simulink model "model1_raw"  (Simulink 7.7)
settings: Solver=VariableStepDiscrete  StartTime=0.0  StopTime=10.0  RelTol=1e-3
values from neighbouring files (symbols this model uses):
  A = A1'    [dyskretny.m]    (also in przebieg.m; zmiennestanu.m)
  C = B1'    [dyskretny.m]    (also in przebieg.m; zmiennestanu.m)
libraries: simulink x3
settings Model: Creator=Andones  LastModifiedBy=qiubix

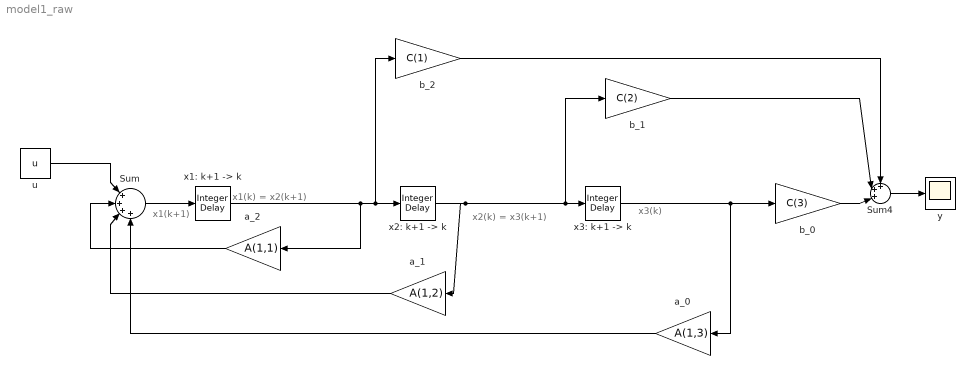
== system model1_raw ==
  note: x1(k+1)
  note: x3(k)
  note: x1(k) = x2(k+1)
  note: x2(k) = x3(k+1)
  " x3: k+1 -> k" : simulink/Discrete/Integer Delay  NumDelays=1  vinit=1  samptime=T_s
  Sum : Sum  Inputs=|++++
  Sum4 : Sum  Inputs=+++|
  a_0 : Gain  Gain=A(1,3)
  a_1 : Gain  Gain=A(1,2)
  a_2 : Gain  Gain=A(1,1)
  b_0 : Gain  Gain=C(3)
  b_1 : Gain  Gain=C(2)
  b_2 : Gain  Gain=C(1)
  u : Constant  Value=u
  "x1: k+1 -> k " : simulink/Discrete/Integer Delay  NumDelays=1  vinit=-1  samptime=T_s
  "x2: k+1 -> k" : simulink/Discrete/Integer Delay  NumDelays=1  vinit=-1  samptime=T_s
  y : Scope
  wires:
  Sum/1 -> "x1: k+1 -> k "/1
  Sum4/1 -> y/1
  b_0/1 -> Sum4/3
  b_1/1 -> Sum4/2
  b_2/1 -> Sum4/1
  "x1: k+1 -> k "/1 -> "x2: k+1 -> k"/1, b_2/1, a_2/1
  "x2: k+1 -> k"/1 -> b_1/1, " x3: k+1 -> k"/1, a_1/1
  a_0/1 -> Sum/4
  a_1/1 -> Sum/3
  " x3: k+1 -> k"/1 -> b_0/1, a_0/1
  u/1 -> Sum/1
  a_2/1 -> Sum/2
